simulink model "simlev"  (R2018a)
settings: Solver=VariableStepAuto  StartTime=0.0  StopTime=30  RelTol=1e-3
undefined symbols (not defined in the file): A, B, M, magnitude
libraries: fuzblock x1
settings Model: Creator=Estudiantes  LastModifiedBy=daniel

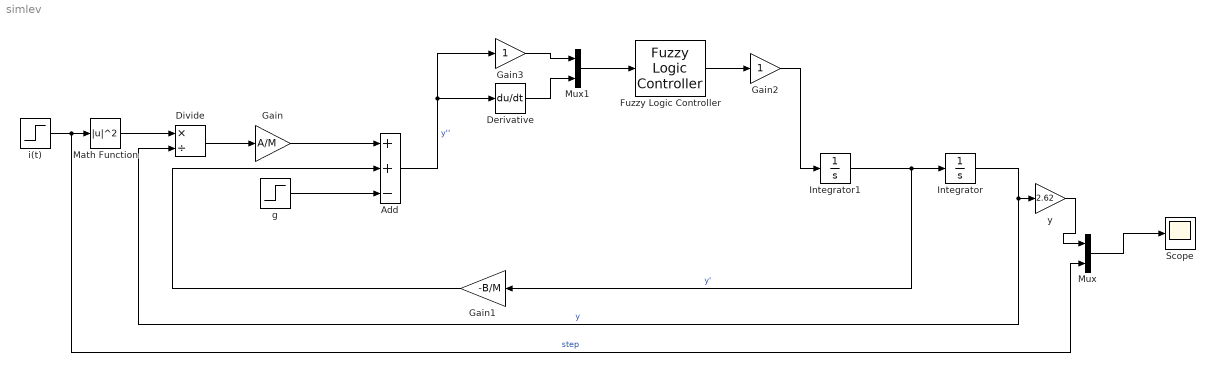
== system simlev ==
  Add : Sum  Inputs=++-
  Derivative : Derivative
  Divide : Product  Inputs=*/
  Fuzzy Logic Controller : fuzblock/Fuzzy Logic  Controller  FIS=sys  OutputSampleNumber=101  DataType=double  FuzzifiedInputs=off  RuleFiringStrengths=off  RuleOutputs=off  AggregatedOutputs=off  SimulateUsing=Interpreted execution  OutOfRangeInputValueMessage=warning  NoRuleFiredMessage=warning  EmptyOutputFuzzySetMessage=warning
  Gain : Gain  Gain=A/M
  Gain1 : Gain  Gain=-B/M
  Gain2 : Gain
  Gain3 : Gain
  Integrator : Integrator
  Integrator1 : Integrator
  Math Function : Math  Operator=magnitude^2  SaturateOnIntegerOverflow=on
  Mux : Mux  Inputs=2
  Mux1 : Mux  Inputs=2
  Scope : Scope
  "g " : Step  After=9.8  SampleTime=0
  "i(t) " : Step  Time=0  SampleTime=0
  y : Gain  Gain=2.62
  wires:
  Add/1 -> Derivative/1, Gain3/1  "y''"
  Integrator1/1 -> Gain1/1, Integrator/1  "y'"
  Integrator/1 -> y/1, Divide/2  "y"
  Gain1/1 -> Add/2
  Mux/1 -> Scope/1
  "g "/1 -> Add/3
  "i(t) "/1 -> Mux/2, Math Function/1  "step"
  Math Function/1 -> Divide/1
  Divide/1 -> Gain/1
  Gain/1 -> Add/1
  Derivative/1 -> Mux1/2
  Gain3/1 -> Mux1/1
  Mux1/1 -> Fuzzy Logic Controller/1
  Fuzzy Logic Controller/1 -> Gain2/1
  Gain2/1 -> Integrator1/1
  y/1 -> Mux/1
